simulink model "frontal"  (R2021b)
settings: Solver=VariableStepAuto  StartTime=0.0  StopTime=2  RelTol=1e-3
values from neighbouring files (symbols this model uses):
  Kx = 1 / tau    (= 6.66666666667)    [inicializarFollowline.m]    (also in inicializarFrontal.m)
  x0 = 0    [inicializarFollowline.m]    (also in inicializarFrontal.m)
  xr = -1    [avaliarFollowline.m]    (also in inicializarFollowline.m = 1; inicializarFrontal.m = 1)
settings Model: Creator=mmaximo  LastModifiedBy=berho
settings SolverCC: AlgebraicLoopSolver=TrustRegion
settings DebuggingCC: SFMachineParentedDataDiag=warning

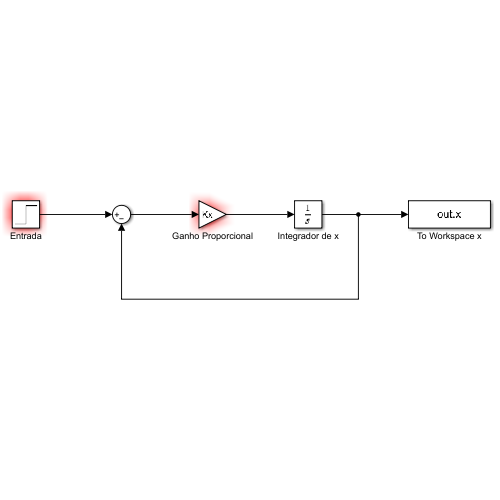
[thumbnail: Simulink's stored preview of the top-level diagram]
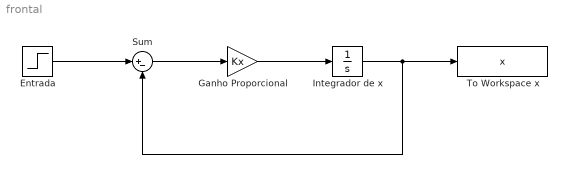
== system frontal ==
  Entrada : Step  Time=0  Before=x0  After=xr  SampleTime=0
  Ganho Proporcional : Gain  Gain=Kx
  Integrador de x : Integrator
  Sum : Sum  Inputs=|+-
  To Workspace x : ToWorkspace  VariableName=x  SaveFormat=Structure With Time  SampleTime=-1
  wires:
  Entrada/1 -> Sum/1
  Integrador de x/1 -> To Workspace x/1, Sum/2
  Sum/1 -> Ganho Proporcional/1
  Ganho Proporcional/1 -> Integrador de x/1
